simulink model "Dyn_Sim"  (Simulink 9.2)
settings: Solver=VariableStepAuto  StartTime=0.0  StopTime=time  FixedStep=0.1  MaxStep=0.1  RelTol=1e-3  EnableMultiTasking=on
values from neighbouring files (symbols this model uses):
  l10d = -3    [runner_simulation.m]
  l1d = in(15)    [control_law1.m]    (also in runner_simulation.m = 2)
  l2d = 1    [runner_simulation.m]
  l3d = 2    [runner_simulation.m]
  l4d = 1    [runner_simulation.m]
  l5d = 3    [runner_simulation.m]
  l6d = -2    [runner_simulation.m]
  l7d = -2    [runner_simulation.m]
  l8d = 5    [runner_simulation.m]
  l9d = -1    [runner_simulation.m]
  q0 = [10 -18 1*pi/2]'    [runner_simulation.m]
  q0_1 = [22 -18 1*pi/2]'    [runner_simulation.m]
  q0_10 = [14 -18 1*pi/2]'    [runner_simulation.m]
  q0_2 = [18.5 -18 1*pi/2]'    [runner_simulation.m]
  q0_3 = [8 -18 1*pi/2]'    [runner_simulation.m]
  q0_4 = [5 -18 1*pi/2]'    [runner_simulation.m]
  q0_5 = [14 -18 1*pi/2]'    [runner_simulation.m]
  q0_6 = [22 -18 1*pi/2]'    [runner_simulation.m]
  q0_7 = [18.5 -18 1*pi/2]'    [runner_simulation.m]
  q0_8 = [8 -18 1*pi/2]'    [runner_simulation.m]
  q0_9 = [5 -18 1*pi/2]'    [runner_simulation.m]
  sai10_d = 3*pi/6+3*pi/2    (= 6.28318530718)    [runner_simulation.m]
  sai1_d = pi/4    (= 0.785398163397)    [runner_simulation.m]
  sai2_d = 2*pi/4    (= 1.57079632679)    [runner_simulation.m]
  sai3_d = -pi/4    (= -0.785398163397)    [runner_simulation.m]
  sai4_d = -2*pi/4    (= -1.57079632679)    [runner_simulation.m]
  sai5_d = 3*pi/6+3*pi/2    (= 6.28318530718)    [runner_simulation.m]
  sai6_d = pi/4    (= 0.785398163397)    [runner_simulation.m]
  sai7_d = -2*pi/8    (= -0.785398163397)    [runner_simulation.m]
  sai8_d = 3*pi/6+3*pi/2    (= 6.28318530718)    [runner_simulation.m]
  sai9_d = 3*pi/6+3*pi/2    (= 6.28318530718)    [runner_simulation.m]
  u0 = [0.1;0.1;0.1]'    [runner_simulation.m]
  u01 = [0;0;0]'    [runner_simulation.m]
Description:
  | Real-Time Van der Pol Simulation
  | 
  | This demonstration shows a real-time version of the Simulink(R) Van der Pol
  | simulation demo. This model does not need any external signals, so it does
  | not need any data acquisition hardware or driver. This makes the model ideal
  | for first experiments with Real-Time Windows Target(TM), without need to
  | worry about proper I/O hardware configuration.
  | 
  | How to run this demo in Normal Mode:
  | 
  | 1) Double-click the orange button to switch to Normal Mode if needed.
  | 2) Start the real-time execution using Simulation->Start.
  | 3) Observe any missed ticks on the Missed Ticks scope.
  | 
  | How to run this demo in External Mode:
  | 
  | 1) Double-click the orange button to switch to External Mode if needed.
  | 2) Build the model using Tools->Code Generation->Build Model.
  | 3) Connect to the real-time code using Simulation->Connect to target.
  | 4) Start the real-time execution using Simulation->Start real-time code.
  | 5) Missed ticks will be always zero.
settings Model: Creator=The MathWorks Inc.  LastModifiedBy=Rasoul  ExtModeTrigDuration=101
settings DataIOCC: SignalLoggingSaveFormat=Dataset  SignalLoggingName=logsOut
settings OptimizationCC: ExpressionDepthLimit=2147483647  InitFltsAndDblsToZero=on  EfficientMapNaN2IntZero=off
settings DebuggingCC: SignalResolutionControl=TryResolveAllWithWarning  AllowSymbolicDim=off
settings HardwareCC: ProdBitPerPointer=64  ProdBitPerSizeT=64  ProdBitPerPtrDiffT=64  ProdLargestAtomicFloat=Float  ProdIntDivRoundTo=Zero  ProdEndianess=LittleEndian  ProdWordSize=64  ProdHWDeviceType=Intel->x86-64 (Windows64)  TargetBitPerLong=64  TargetBitPerPointer=64  TargetIntDivRoundTo=Zero  TargetEndianess=LittleEndian  TargetWordSize=64  TargetHWDeviceType=Intel->x86-64
settings RTWCC: SystemTargetFile=sldrt.tlc  TemplateMakefile=sldrt.tmf  Description=Simulink Desktop Real-Time  RTWCompilerOptimization=on
settings CodeAppCC: MaxIdLength=95
settings SimulinkDesktopRealTimeCC: TargetPreCompLibLocation=C:\Program Files\MATLAB\R2018b\toolbox\sldrt\lib\win64  TargetLangStandard=C89/C90 (ANSI)  SupportVariableSizeSignals=off  PreserveStateflowLocalDataDimensions=off

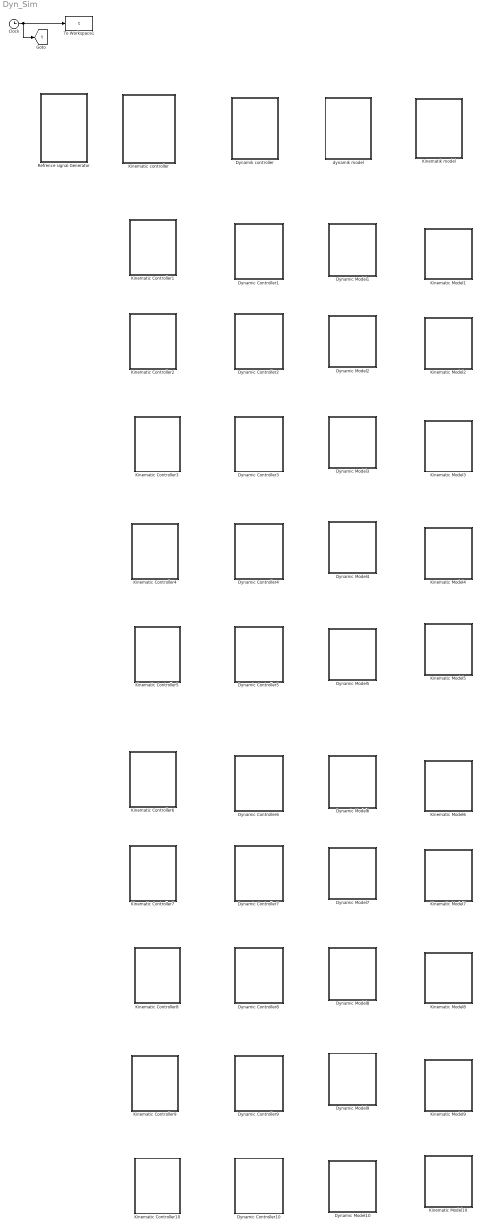
== system Dyn_Sim ==
  Clock : Clock
  Dynamic Controller1 : Subsystem
  Dynamic Controller10 : Subsystem
  Dynamic Controller2 : Subsystem
  Dynamic Controller3 : Subsystem
  Dynamic Controller4 : Subsystem
  Dynamic Controller5 : Subsystem
  Dynamic Controller6 : Subsystem
  Dynamic Controller7 : Subsystem
  Dynamic Controller8 : Subsystem
  Dynamic Controller9 : Subsystem
  Dynamic Model1 : Subsystem
  Dynamic Model10 : Subsystem
  Dynamic Model2 : Subsystem
  Dynamic Model3 : Subsystem
  Dynamic Model4 : Subsystem
  Dynamic Model5 : Subsystem
  Dynamic Model6 : Subsystem
  Dynamic Model7 : Subsystem
  Dynamic Model8 : Subsystem
  Dynamic Model9 : Subsystem
  Dynamik controller : Subsystem
  Kinematic Controller1 : Subsystem
  Kinematic Controller10 : Subsystem
  Kinematic Controller2 : Subsystem
  Kinematic Controller3 : Subsystem
  Kinematic Controller4 : Subsystem
  Kinematic Controller5 : Subsystem
  Kinematic Controller6 : Subsystem
  Kinematic Controller7 : Subsystem
  Kinematic Controller8 : Subsystem
  Kinematic Controller9 : Subsystem
  Kinematic Model1 : Subsystem
  Kinematic Model10 : Subsystem
  Kinematic Model2 : Subsystem
  Kinematic Model3 : Subsystem
  Kinematic Model4 : Subsystem
  Kinematic Model5 : Subsystem
  Kinematic Model6 : Subsystem
  Kinematic Model7 : Subsystem
  Kinematic Model8 : Subsystem
  Kinematic Model9 : Subsystem
  Kinematic controller : Subsystem
  Kinematik model : Subsystem
  "Refrence signal Generator " : Subsystem
  To Workspace1 : ToWorkspace  VariableName=t  SampleTime=-1
  dynamik model : Subsystem
  tag scope: t=global
  wires:
  Clock/1 -> To Workspace1/1, [t]

== system Dyn_Sim/Dynamic Controller1 ==
  Demux1 : Demux  Outputs=2
  Demux2 : Demux  Outputs=3
  Demux4 : Demux  Outputs=3
  Mux4 : Mux  Inputs=3
  Mux7 : Mux
  Mux8 : Mux  Inputs=3
  Scope10 : Scope
  Scope9 : Scope
  To Workspace12 : ToWorkspace  VariableName=tau1  SampleTime=-1
  dynamic_control : MATLABFcn  MATLABFcn=dynamic_control  OutputDimensions=6  OutputSignalType=real
  tag scope: tau1=global
  wires:
  Mux4/1 -> Scope9/1, To Workspace12/1, [tau1]
  Mux7/1 -> dynamic_control/1
  [duc1] -> Mux7/3
  Mux8/1 -> Scope10/1
  Demux4/1 -> Mux4/1
  [t] -> Mux7/4
  [uu1] -> Mux7/1
  [uc1] -> Mux7/2
  dynamic_control/1 -> Demux1/1
  Demux4/2 -> Mux4/2
  Demux1/1 -> Demux4/1
  Demux1/2 -> Demux2/1
  Demux2/1 -> Mux8/1
  Demux2/2 -> Mux8/2
  Demux4/3 -> Mux4/3
  Demux2/3 -> Mux8/3

== system Dyn_Sim/Dynamic Controller10 ==
  Demux1 : Demux  Outputs=2
  Demux2 : Demux  Outputs=3
  Demux4 : Demux  Outputs=3
  Mux4 : Mux  Inputs=3
  Mux7 : Mux
  Mux8 : Mux  Inputs=3
  Scope10 : Scope
  Scope9 : Scope
  To Workspace12 : ToWorkspace  VariableName=tau10  SampleTime=-1
  dynamic_control : MATLABFcn  MATLABFcn=dynamic_control  OutputDimensions=6  OutputSignalType=real
  tag scope: tau10=global
  wires:
  Demux2/3 -> Mux8/3
  Demux4/3 -> Mux4/3
  Demux2/2 -> Mux8/2
  Demux2/1 -> Mux8/1
  Demux1/2 -> Demux2/1
  Demux1/1 -> Demux4/1
  Demux4/2 -> Mux4/2
  dynamic_control/1 -> Demux1/1
  [uc10] -> Mux7/2
  [uu10] -> Mux7/1
  [t] -> Mux7/4
  Demux4/1 -> Mux4/1
  Mux8/1 -> Scope10/1
  [duc10] -> Mux7/3
  Mux7/1 -> dynamic_control/1
  Mux4/1 -> [tau10], To Workspace12/1, Scope9/1

== system Dyn_Sim/Dynamic Controller2 ==
  Demux1 : Demux  Outputs=2
  Demux2 : Demux  Outputs=3
  Demux4 : Demux  Outputs=3
  Mux4 : Mux  Inputs=3
  Mux7 : Mux
  Mux8 : Mux  Inputs=3
  Scope10 : Scope
  Scope9 : Scope
  To Workspace12 : ToWorkspace  VariableName=tau2  SampleTime=-1
  dynamic_control : MATLABFcn  MATLABFcn=dynamic_control  OutputDimensions=6  OutputSignalType=real
  tag scope: tau2=global
  wires:
  Demux2/3 -> Mux8/3
  Demux4/3 -> Mux4/3
  Demux2/1 -> Mux8/1
  Demux4/1 -> Mux4/1
  Mux8/1 -> Scope10/1
  Demux2/2 -> Mux8/2
  [duc2] -> Mux7/3
  dynamic_control/1 -> Demux1/1
  [t] -> Mux7/4
  Demux1/2 -> Demux2/1
  Demux4/2 -> Mux4/2
  [uu2] -> Mux7/1
  Demux1/1 -> Demux4/1
  Mux7/1 -> dynamic_control/1
  [uc2] -> Mux7/2
  Mux4/1 -> [tau2], To Workspace12/1, Scope9/1

== system Dyn_Sim/Dynamic Controller3 ==
  Demux1 : Demux  Outputs=2
  Demux2 : Demux  Outputs=3
  Demux4 : Demux  Outputs=3
  Mux4 : Mux  Inputs=3
  Mux7 : Mux
  Mux8 : Mux  Inputs=3
  Scope10 : Scope
  Scope9 : Scope
  To Workspace12 : ToWorkspace  VariableName=tau3  SampleTime=-1
  dynamic_control : MATLABFcn  MATLABFcn=dynamic_control  OutputDimensions=6  OutputSignalType=real
  tag scope: tau3=global
  wires:
  Mux4/1 -> Scope9/1, To Workspace12/1, [tau3]
  Mux7/1 -> dynamic_control/1
  [duc3] -> Mux7/3
  Mux8/1 -> Scope10/1
  Demux4/1 -> Mux4/1
  [t] -> Mux7/4
  [uu3] -> Mux7/1
  [uc3] -> Mux7/2
  dynamic_control/1 -> Demux1/1
  Demux4/2 -> Mux4/2
  Demux1/1 -> Demux4/1
  Demux1/2 -> Demux2/1
  Demux2/1 -> Mux8/1
  Demux2/2 -> Mux8/2
  Demux4/3 -> Mux4/3
  Demux2/3 -> Mux8/3

== system Dyn_Sim/Dynamic Controller4 ==
  Demux1 : Demux  Outputs=2
  Demux2 : Demux  Outputs=3
  Demux4 : Demux  Outputs=3
  Mux4 : Mux  Inputs=3
  Mux7 : Mux
  Mux8 : Mux  Inputs=3
  Scope10 : Scope
  Scope9 : Scope
  To Workspace12 : ToWorkspace  VariableName=tau4  SampleTime=-1
  dynamic_control : MATLABFcn  MATLABFcn=dynamic_control  OutputDimensions=6  OutputSignalType=real
  tag scope: tau4=global
  wires:
  Mux4/1 -> Scope9/1, To Workspace12/1, [tau4]
  Mux7/1 -> dynamic_control/1
  [duc4] -> Mux7/3
  Mux8/1 -> Scope10/1
  Demux4/1 -> Mux4/1
  [t] -> Mux7/4
  [uu4] -> Mux7/1
  [uc4] -> Mux7/2
  dynamic_control/1 -> Demux1/1
  Demux4/2 -> Mux4/2
  Demux1/1 -> Demux4/1
  Demux1/2 -> Demux2/1
  Demux2/1 -> Mux8/1
  Demux2/2 -> Mux8/2
  Demux4/3 -> Mux4/3
  Demux2/3 -> Mux8/3

== system Dyn_Sim/Dynamic Controller5 ==
  Demux1 : Demux  Outputs=2
  Demux2 : Demux  Outputs=3
  Demux4 : Demux  Outputs=3
  Mux4 : Mux  Inputs=3
  Mux7 : Mux
  Mux8 : Mux  Inputs=3
  Scope10 : Scope
  Scope9 : Scope
  To Workspace12 : ToWorkspace  VariableName=tau5  SampleTime=-1
  dynamic_control : MATLABFcn  MATLABFcn=dynamic_control  OutputDimensions=6  OutputSignalType=real
  tag scope: tau5=global
  wires:
  Mux4/1 -> Scope9/1, To Workspace12/1, [tau5]
  Mux7/1 -> dynamic_control/1
  [duc5] -> Mux7/3
  Mux8/1 -> Scope10/1
  Demux4/1 -> Mux4/1
  [t] -> Mux7/4
  [uu5] -> Mux7/1
  [uc5] -> Mux7/2
  dynamic_control/1 -> Demux1/1
  Demux4/2 -> Mux4/2
  Demux1/1 -> Demux4/1
  Demux1/2 -> Demux2/1
  Demux2/1 -> Mux8/1
  Demux2/2 -> Mux8/2
  Demux4/3 -> Mux4/3
  Demux2/3 -> Mux8/3

== system Dyn_Sim/Dynamic Controller6 ==
  Demux1 : Demux  Outputs=2
  Demux2 : Demux  Outputs=3
  Demux4 : Demux  Outputs=3
  Mux4 : Mux  Inputs=3
  Mux7 : Mux
  Mux8 : Mux  Inputs=3
  Scope10 : Scope
  Scope9 : Scope
  To Workspace12 : ToWorkspace  VariableName=tau6  SampleTime=-1
  dynamic_control : MATLABFcn  MATLABFcn=dynamic_control  OutputDimensions=6  OutputSignalType=real
  tag scope: tau6=global
  wires:
  Demux2/3 -> Mux8/3
  Demux4/3 -> Mux4/3
  Demux2/2 -> Mux8/2
  Demux2/1 -> Mux8/1
  Demux1/2 -> Demux2/1
  Demux1/1 -> Demux4/1
  Demux4/2 -> Mux4/2
  dynamic_control/1 -> Demux1/1
  [uc6] -> Mux7/2
  [uu6] -> Mux7/1
  [t] -> Mux7/4
  Demux4/1 -> Mux4/1
  Mux8/1 -> Scope10/1
  [duc6] -> Mux7/3
  Mux7/1 -> dynamic_control/1
  Mux4/1 -> [tau6], To Workspace12/1, Scope9/1

== system Dyn_Sim/Dynamic Controller7 ==
  Demux1 : Demux  Outputs=2
  Demux2 : Demux  Outputs=3
  Demux4 : Demux  Outputs=3
  Mux4 : Mux  Inputs=3
  Mux7 : Mux
  Mux8 : Mux  Inputs=3
  Scope10 : Scope
  Scope9 : Scope
  To Workspace12 : ToWorkspace  VariableName=tau7  SampleTime=-1
  dynamic_control : MATLABFcn  MATLABFcn=dynamic_control  OutputDimensions=6  OutputSignalType=real
  tag scope: tau7=global
  wires:
  Mux4/1 -> Scope9/1, To Workspace12/1, [tau7]
  [uc7] -> Mux7/2
  Mux7/1 -> dynamic_control/1
  Demux1/1 -> Demux4/1
  [uu7] -> Mux7/1
  Demux4/2 -> Mux4/2
  Demux1/2 -> Demux2/1
  [t] -> Mux7/4
  dynamic_control/1 -> Demux1/1
  [duc7] -> Mux7/3
  Demux2/2 -> Mux8/2
  Mux8/1 -> Scope10/1
  Demux4/1 -> Mux4/1
  Demux2/1 -> Mux8/1
  Demux4/3 -> Mux4/3
  Demux2/3 -> Mux8/3

== system Dyn_Sim/Dynamic Controller8 ==
  Demux1 : Demux  Outputs=2
  Demux2 : Demux  Outputs=3
  Demux4 : Demux  Outputs=3
  Mux4 : Mux  Inputs=3
  Mux7 : Mux
  Mux8 : Mux  Inputs=3
  Scope10 : Scope
  Scope9 : Scope
  To Workspace12 : ToWorkspace  VariableName=tau8  SampleTime=-1
  dynamic_control : MATLABFcn  MATLABFcn=dynamic_control  OutputDimensions=6  OutputSignalType=real
  tag scope: tau8=global
  wires:
  Demux2/3 -> Mux8/3
  Demux4/3 -> Mux4/3
  Demux2/2 -> Mux8/2
  Demux2/1 -> Mux8/1
  Demux1/2 -> Demux2/1
  Demux1/1 -> Demux4/1
  Demux4/2 -> Mux4/2
  dynamic_control/1 -> Demux1/1
  [uc8] -> Mux7/2
  [uu8] -> Mux7/1
  [t] -> Mux7/4
  Demux4/1 -> Mux4/1
  Mux8/1 -> Scope10/1
  [duc8] -> Mux7/3
  Mux7/1 -> dynamic_control/1
  Mux4/1 -> [tau8], To Workspace12/1, Scope9/1

== system Dyn_Sim/Dynamic Controller9 ==
  Demux1 : Demux  Outputs=2
  Demux2 : Demux  Outputs=3
  Demux4 : Demux  Outputs=3
  Mux4 : Mux  Inputs=3
  Mux7 : Mux
  Mux8 : Mux  Inputs=3
  Scope10 : Scope
  Scope9 : Scope
  To Workspace12 : ToWorkspace  VariableName=tau9  SampleTime=-1
  dynamic_control : MATLABFcn  MATLABFcn=dynamic_control  OutputDimensions=6  OutputSignalType=real
  tag scope: tau9=global
  wires:
  Demux2/3 -> Mux8/3
  Demux4/3 -> Mux4/3
  Demux2/2 -> Mux8/2
  Demux2/1 -> Mux8/1
  Demux1/2 -> Demux2/1
  Demux1/1 -> Demux4/1
  Demux4/2 -> Mux4/2
  dynamic_control/1 -> Demux1/1
  [uc9] -> Mux7/2
  [uu9] -> Mux7/1
  [t] -> Mux7/4
  Demux4/1 -> Mux4/1
  Mux8/1 -> Scope10/1
  [duc9] -> Mux7/3
  Mux7/1 -> dynamic_control/1
  Mux4/1 -> [tau9], To Workspace12/1, Scope9/1

== system Dyn_Sim/Dynamic Model1 ==
  Integrator2 : Integrator  InitialCondition=u01
  Mux9 : Mux  Inputs=3
  To Workspace11 : ToWorkspace  VariableName=uu1  SampleTime=-1
  dynamic_model : MATLABFcn  MATLABFcn=dynamic_model  OutputDimensions=3  OutputSignalType=real
  tag scope: uu1=global
  wires:
  [tau1] -> Mux9/2
  [uu1] -> Mux9/1
  dynamic_model/1 -> Integrator2/1
  Mux9/1 -> dynamic_model/1
  [t] -> Mux9/3
  Integrator2/1 -> [uu1], To Workspace11/1

== system Dyn_Sim/Dynamic Model10 ==
  Integrator2 : Integrator  InitialCondition=u01
  Mux9 : Mux  Inputs=3
  To Workspace11 : ToWorkspace  VariableName=uu10  SampleTime=-1
  dynamic_model : MATLABFcn  MATLABFcn=dynamic_model  OutputDimensions=3  OutputSignalType=real
  tag scope: uu10=global
  wires:
  Integrator2/1 -> To Workspace11/1, [uu10]
  [t] -> Mux9/3
  Mux9/1 -> dynamic_model/1
  dynamic_model/1 -> Integrator2/1
  [uu10] -> Mux9/1
  [tau10] -> Mux9/2

== system Dyn_Sim/Dynamic Model2 ==
  Integrator2 : Integrator  InitialCondition=u01
  Mux9 : Mux  Inputs=3
  To Workspace11 : ToWorkspace  VariableName=uu2  SampleTime=-1
  dynamic_model : MATLABFcn  MATLABFcn=dynamic_model  OutputDimensions=3  OutputSignalType=real
  tag scope: uu2=global
  wires:
  Mux9/1 -> dynamic_model/1
  [tau2] -> Mux9/2
  dynamic_model/1 -> Integrator2/1
  Integrator2/1 -> To Workspace11/1, [uu2]
  [t] -> Mux9/3
  [uu2] -> Mux9/1

== system Dyn_Sim/Dynamic Model3 ==
  Integrator2 : Integrator  InitialCondition=u01
  Mux9 : Mux  Inputs=3
  To Workspace11 : ToWorkspace  VariableName=uu3  SampleTime=-1
  dynamic_model : MATLABFcn  MATLABFcn=dynamic_model  OutputDimensions=3  OutputSignalType=real
  tag scope: uu3=global
  wires:
  [tau3] -> Mux9/2
  [uu3] -> Mux9/1
  dynamic_model/1 -> Integrator2/1
  Mux9/1 -> dynamic_model/1
  [t] -> Mux9/3
  Integrator2/1 -> [uu3], To Workspace11/1

== system Dyn_Sim/Dynamic Model4 ==
  Integrator2 : Integrator  InitialCondition=u01
  Mux9 : Mux  Inputs=3
  To Workspace11 : ToWorkspace  VariableName=uu4  SampleTime=-1
  dynamic_model : MATLABFcn  MATLABFcn=dynamic_model  OutputDimensions=3  OutputSignalType=real
  tag scope: uu4=global
  wires:
  [tau4] -> Mux9/2
  [uu4] -> Mux9/1
  dynamic_model/1 -> Integrator2/1
  Mux9/1 -> dynamic_model/1
  [t] -> Mux9/3
  Integrator2/1 -> [uu4], To Workspace11/1

== system Dyn_Sim/Dynamic Model5 ==
  Integrator2 : Integrator  InitialCondition=u01
  Mux9 : Mux  Inputs=3
  To Workspace11 : ToWorkspace  VariableName=uu5  SampleTime=-1
  dynamic_model : MATLABFcn  MATLABFcn=dynamic_model  OutputDimensions=3  OutputSignalType=real
  tag scope: uu5=global
  wires:
  [tau5] -> Mux9/2
  [uu5] -> Mux9/1
  dynamic_model/1 -> Integrator2/1
  Mux9/1 -> dynamic_model/1
  [t] -> Mux9/3
  Integrator2/1 -> [uu5], To Workspace11/1

== system Dyn_Sim/Dynamic Model6 ==
  Integrator2 : Integrator  InitialCondition=u01
  Mux9 : Mux  Inputs=3
  To Workspace11 : ToWorkspace  VariableName=uu6  SampleTime=-1
  dynamic_model : MATLABFcn  MATLABFcn=dynamic_model  OutputDimensions=3  OutputSignalType=real
  tag scope: uu6=global
  wires:
  Integrator2/1 -> To Workspace11/1, [uu6]
  [t] -> Mux9/3
  Mux9/1 -> dynamic_model/1
  dynamic_model/1 -> Integrator2/1
  [uu6] -> Mux9/1
  [tau6] -> Mux9/2

== system Dyn_Sim/Dynamic Model7 ==
  Integrator2 : Integrator  InitialCondition=u01
  Mux9 : Mux  Inputs=3
  To Workspace11 : ToWorkspace  VariableName=uu7  SampleTime=-1
  dynamic_model : MATLABFcn  MATLABFcn=dynamic_model  OutputDimensions=3  OutputSignalType=real
  tag scope: uu7=global
  wires:
  [uu7] -> Mux9/1
  [t] -> Mux9/3
  Integrator2/1 -> [uu7], To Workspace11/1
  dynamic_model/1 -> Integrator2/1
  [tau7] -> Mux9/2
  Mux9/1 -> dynamic_model/1

== system Dyn_Sim/Dynamic Model8 ==
  Integrator2 : Integrator  InitialCondition=u01
  Mux9 : Mux  Inputs=3
  To Workspace11 : ToWorkspace  VariableName=uu8  SampleTime=-1
  dynamic_model : MATLABFcn  MATLABFcn=dynamic_model  OutputDimensions=3  OutputSignalType=real
  tag scope: uu8=global
  wires:
  Integrator2/1 -> To Workspace11/1, [uu8]
  [t] -> Mux9/3
  Mux9/1 -> dynamic_model/1
  dynamic_model/1 -> Integrator2/1
  [uu8] -> Mux9/1
  [tau8] -> Mux9/2

== system Dyn_Sim/Dynamic Model9 ==
  Integrator2 : Integrator  InitialCondition=u01
  Mux9 : Mux  Inputs=3
  To Workspace11 : ToWorkspace  VariableName=uu9  SampleTime=-1
  dynamic_model : MATLABFcn  MATLABFcn=dynamic_model  OutputDimensions=3  OutputSignalType=real
  tag scope: uu9=global
  wires:
  Integrator2/1 -> To Workspace11/1, [uu9]
  [t] -> Mux9/3
  Mux9/1 -> dynamic_model/1
  dynamic_model/1 -> Integrator2/1
  [uu9] -> Mux9/1
  [tau9] -> Mux9/2

== system Dyn_Sim/Dynamik controller ==
  Demux4 : Demux  Outputs=6
  Mux4 : Mux  Inputs=3
  Mux7 : Mux
  Mux8 : Mux  Inputs=3
  Scope10 : Scope
  Scope9 : Scope
  To Workspace12 : ToWorkspace  VariableName=tau  SampleTime=-1
  dynamic_control : MATLABFcn  MATLABFcn=dynamic_control  OutputDimensions=6  OutputSignalType=real
  tag scope: tau=global
  wires:
  Demux4/6 -> Mux8/3
  Demux4/5 -> Mux8/2
  Demux4/3 -> Mux4/3
  Mux4/1 -> To Workspace12/1, Scope9/1, [tau]
  dynamic_control/1 -> Demux4/1
  [uu] -> Mux7/1
  Mux8/1 -> Scope10/1
  Demux4/4 -> Mux8/1
  [duc] -> Mux7/3
  [uc] -> Mux7/2
  Demux4/1 -> Mux4/1
  Demux4/2 -> Mux4/2
  Mux7/1 -> dynamic_control/1
  [t] -> Mux7/4

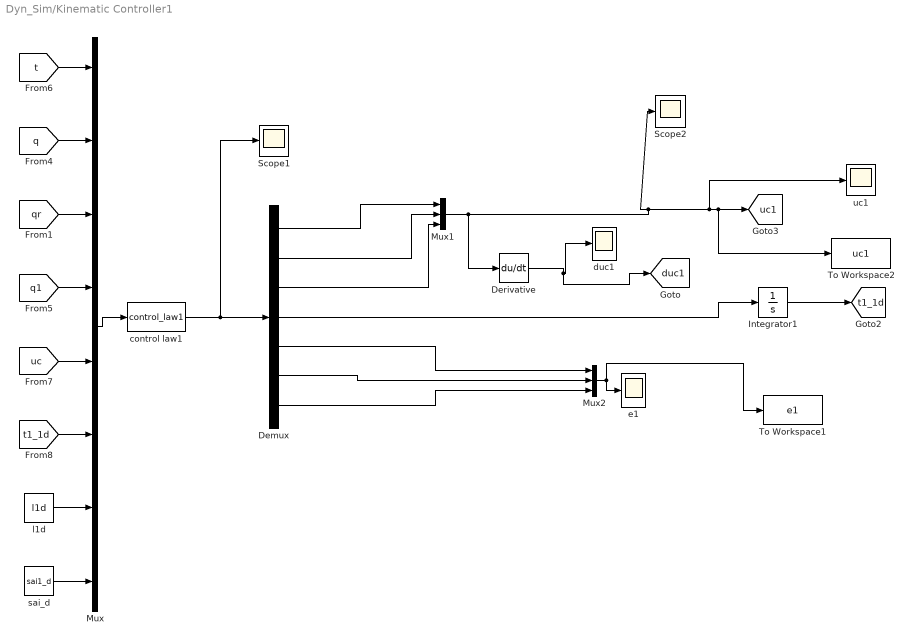
== system Dyn_Sim/Kinematic Controller1 ==
  Demux : Demux  Outputs=7
  Derivative : Derivative
  Integrator1 : Integrator  InitialCondition=pi/2
  Mux : Mux  Inputs=8
  Mux1 : Mux  Inputs=3
  Mux2 : Mux  Inputs=3
  Scope1 : Scope
  Scope2 : Scope
  To Workspace1 : ToWorkspace  VariableName=e1  SampleTime=-1
  To Workspace2 : ToWorkspace  VariableName=uc1  SampleTime=-1
  control law1 : MATLABFcn  MATLABFcn=control_law1  OutputDimensions=7  OutputSignalType=real
  duc1 : Scope
  e1 : Scope
  l1d : Constant  Value=l1d
  sai_d : Constant  Value=sai1_d
  uc1 : Scope
  tag scope: duc1=global, t1_1d=global, uc1=global
  wires:
  control law1/1 -> Scope1/1, Demux/1
  Mux/1 -> control law1/1
  Integrator1/1 -> [t1_1d]
  Mux1/1 -> Derivative/1, uc1/1, To Workspace2/1, [uc1], Scope2/1
  Demux/1 -> Mux1/1
  Demux/2 -> Mux1/2
  Mux2/1 -> e1/1, To Workspace1/1
  Derivative/1 -> [duc1], duc1/1
  [uc] -> Mux/5
  [q1] -> Mux/4
  [qr] -> Mux/3
  [q] -> Mux/2
  [t] -> Mux/1
  [t1_1d] -> Mux/6
  l1d/1 -> Mux/7
  sai_d/1 -> Mux/8
  Demux/3 -> Mux1/3
  Demux/4 -> Integrator1/1
  Demux/5 -> Mux2/1
  Demux/6 -> Mux2/2
  Demux/7 -> Mux2/3

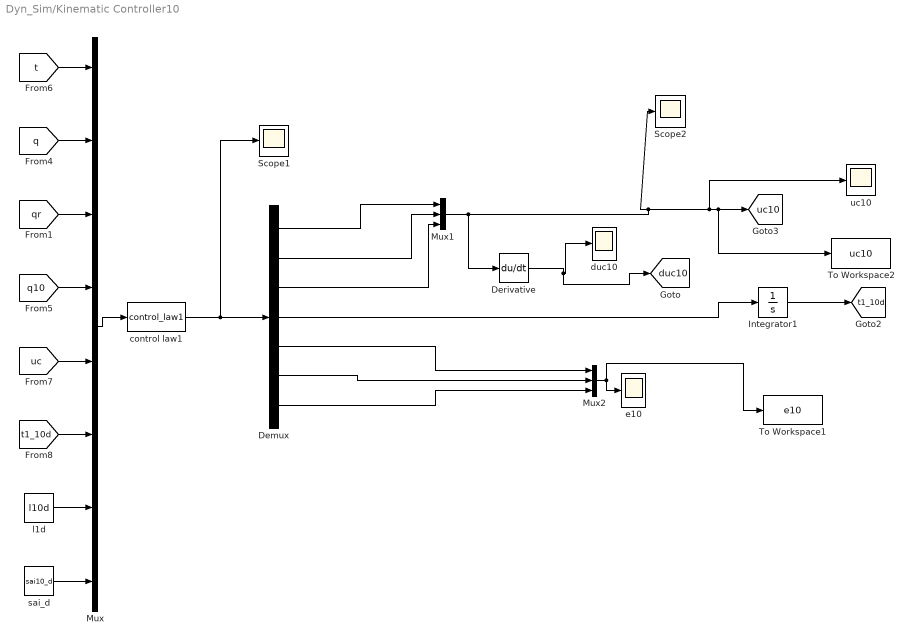
== system Dyn_Sim/Kinematic Controller10 ==
  Demux : Demux  Outputs=7
  Derivative : Derivative
  Integrator1 : Integrator  InitialCondition=pi/2
  Mux : Mux  Inputs=8
  Mux1 : Mux  Inputs=3
  Mux2 : Mux  Inputs=3
  Scope1 : Scope
  Scope2 : Scope
  To Workspace1 : ToWorkspace  VariableName=e10  SampleTime=-1
  To Workspace2 : ToWorkspace  VariableName=uc10  SampleTime=-1
  control law1 : MATLABFcn  MATLABFcn=control_law1  OutputDimensions=7  OutputSignalType=real
  duc10 : Scope
  "e10 " : Scope
  l1d : Constant  Value=l10d
  sai_d : Constant  Value=sai10_d
  uc10 : Scope
  tag scope: duc10=global, t1_10d=global, uc10=global
  wires:
  Demux/7 -> Mux2/3
  Demux/6 -> Mux2/2
  Demux/5 -> Mux2/1
  Demux/4 -> Integrator1/1
  Demux/3 -> Mux1/3
  sai_d/1 -> Mux/8
  l1d/1 -> Mux/7
  [t1_10d] -> Mux/6
  [t] -> Mux/1
  [q] -> Mux/2
  [qr] -> Mux/3
  [q10] -> Mux/4
  [uc] -> Mux/5
  Derivative/1 -> duc10/1, [duc10]
  Mux2/1 -> To Workspace1/1, "e10 "/1
  Demux/2 -> Mux1/2
  Demux/1 -> Mux1/1
  Mux1/1 -> Scope2/1, [uc10], To Workspace2/1, uc10/1, Derivative/1
  Integrator1/1 -> [t1_10d]
  Mux/1 -> control law1/1
  control law1/1 -> Demux/1, Scope1/1

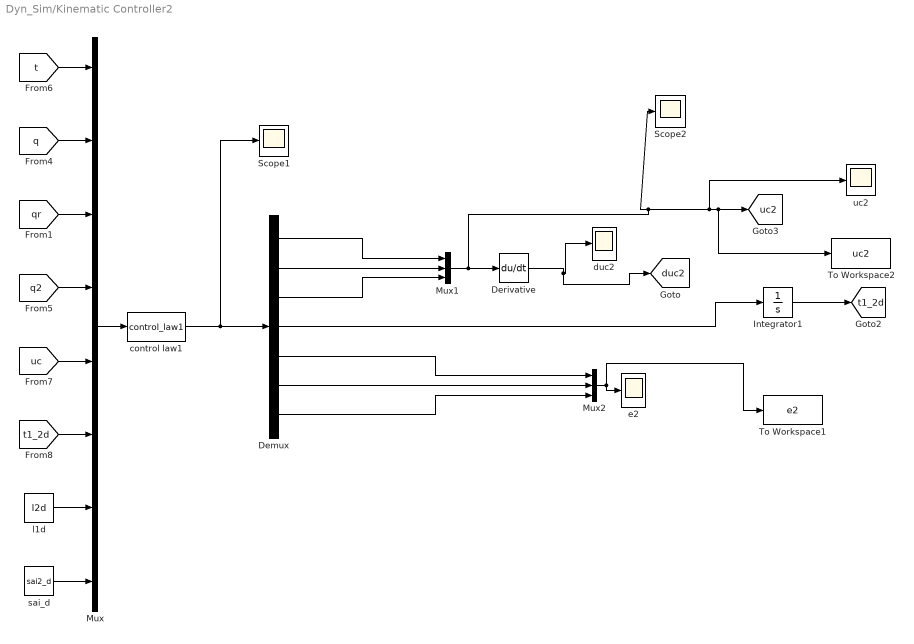
== system Dyn_Sim/Kinematic Controller2 ==
  Demux : Demux  Outputs=7
  Derivative : Derivative
  Integrator1 : Integrator  InitialCondition=pi/2
  Mux : Mux  Inputs=8
  Mux1 : Mux  Inputs=3
  Mux2 : Mux  Inputs=3
  Scope1 : Scope
  Scope2 : Scope
  To Workspace1 : ToWorkspace  VariableName=e2  SampleTime=-1
  To Workspace2 : ToWorkspace  VariableName=uc2  SampleTime=-1
  control law1 : MATLABFcn  MATLABFcn=control_law1  OutputDimensions=7  OutputSignalType=real
  duc2 : Scope
  e2 : Scope
  l1d : Constant  Value=l2d
  sai_d : Constant  Value=sai2_d
  uc2 : Scope
  tag scope: duc2=global, t1_2d=global, uc2=global
  wires:
  Mux/1 -> control law1/1
  control law1/1 -> Demux/1, Scope1/1
  Mux1/1 -> Scope2/1, [uc2], To Workspace2/1, uc2/1, Derivative/1
  Integrator1/1 -> [t1_2d]
  Demux/1 -> Mux1/1
  [q2] -> Mux/4
  Demux/2 -> Mux1/2
  Derivative/1 -> duc2/1, [duc2]
  [t] -> Mux/1
  [uc] -> Mux/5
  [qr] -> Mux/3
  [q] -> Mux/2
  Mux2/1 -> To Workspace1/1, e2/1
  [t1_2d] -> Mux/6
  l1d/1 -> Mux/7
  sai_d/1 -> Mux/8
  Demux/3 -> Mux1/3
  Demux/4 -> Integrator1/1
  Demux/5 -> Mux2/1
  Demux/6 -> Mux2/2
  Demux/7 -> Mux2/3

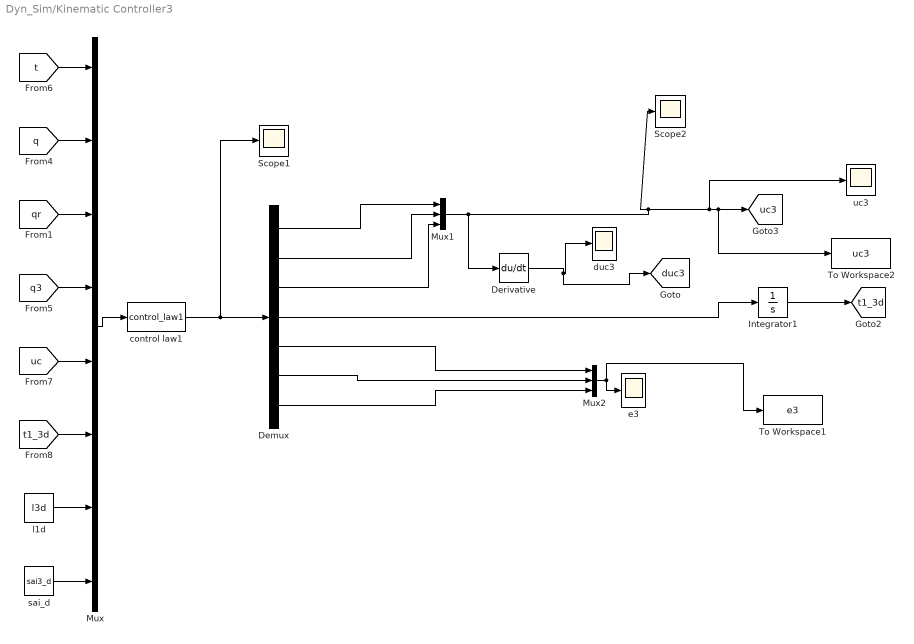
== system Dyn_Sim/Kinematic Controller3 ==
  Demux : Demux  Outputs=7
  Derivative : Derivative
  Integrator1 : Integrator  InitialCondition=pi/2
  Mux : Mux  Inputs=8
  Mux1 : Mux  Inputs=3
  Mux2 : Mux  Inputs=3
  Scope1 : Scope
  Scope2 : Scope
  To Workspace1 : ToWorkspace  VariableName=e3  SampleTime=-1
  To Workspace2 : ToWorkspace  VariableName=uc3  SampleTime=-1
  control law1 : MATLABFcn  MATLABFcn=control_law1  OutputDimensions=7  OutputSignalType=real
  duc3 : Scope
  e3 : Scope
  l1d : Constant  Value=l3d
  sai_d : Constant  Value=sai3_d
  uc3 : Scope
  tag scope: duc3=global, t1_3d=global, uc3=global
  wires:
  control law1/1 -> Scope1/1, Demux/1
  Mux/1 -> control law1/1
  Integrator1/1 -> [t1_3d]
  Mux1/1 -> Derivative/1, uc3/1, To Workspace2/1, [uc3], Scope2/1
  Demux/1 -> Mux1/1
  Demux/2 -> Mux1/2
  Mux2/1 -> e3/1, To Workspace1/1
  Derivative/1 -> [duc3], duc3/1
  [uc] -> Mux/5
  [q3] -> Mux/4
  [qr] -> Mux/3
  [q] -> Mux/2
  [t] -> Mux/1
  [t1_3d] -> Mux/6
  l1d/1 -> Mux/7
  sai_d/1 -> Mux/8
  Demux/3 -> Mux1/3
  Demux/4 -> Integrator1/1
  Demux/5 -> Mux2/1
  Demux/6 -> Mux2/2
  Demux/7 -> Mux2/3

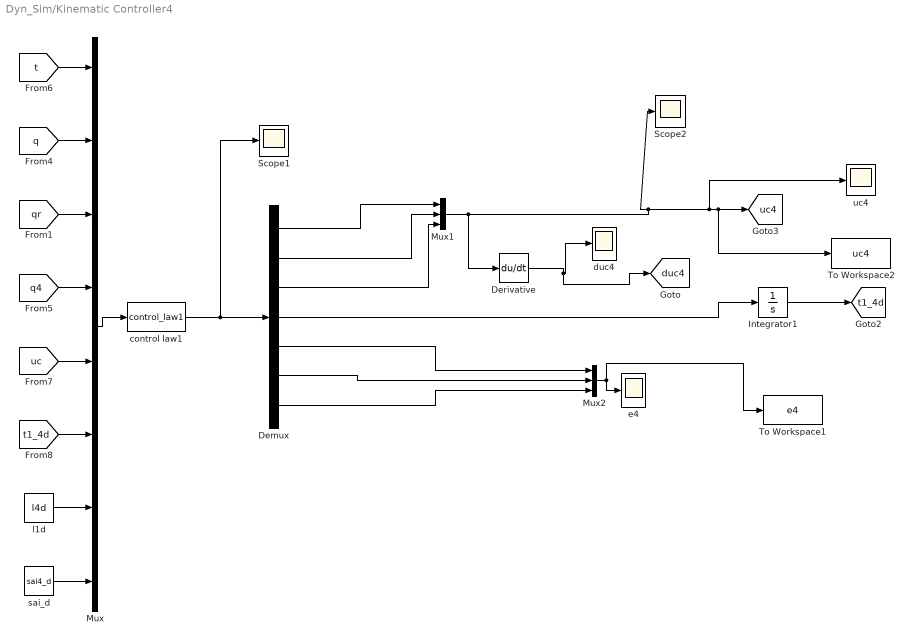
== system Dyn_Sim/Kinematic Controller4 ==
  Demux : Demux  Outputs=7
  Derivative : Derivative
  Integrator1 : Integrator  InitialCondition=pi/2
  Mux : Mux  Inputs=8
  Mux1 : Mux  Inputs=3
  Mux2 : Mux  Inputs=3
  Scope1 : Scope
  Scope2 : Scope
  To Workspace1 : ToWorkspace  VariableName=e4  SampleTime=-1
  To Workspace2 : ToWorkspace  VariableName=uc4  SampleTime=-1
  control law1 : MATLABFcn  MATLABFcn=control_law1  OutputDimensions=7  OutputSignalType=real
  duc4 : Scope
  e4 : Scope
  l1d : Constant  Value=l4d
  sai_d : Constant  Value=sai4_d
  uc4 : Scope
  tag scope: duc4=global, t1_4d=global, uc4=global
  wires:
  control law1/1 -> Scope1/1, Demux/1
  Mux/1 -> control law1/1
  Integrator1/1 -> [t1_4d]
  Mux1/1 -> Derivative/1, uc4/1, To Workspace2/1, [uc4], Scope2/1
  Demux/1 -> Mux1/1
  Demux/2 -> Mux1/2
  Mux2/1 -> e4/1, To Workspace1/1
  Derivative/1 -> [duc4], duc4/1
  [uc] -> Mux/5
  [q4] -> Mux/4
  [qr] -> Mux/3
  [q] -> Mux/2
  [t] -> Mux/1
  [t1_4d] -> Mux/6
  l1d/1 -> Mux/7
  sai_d/1 -> Mux/8
  Demux/3 -> Mux1/3
  Demux/4 -> Integrator1/1
  Demux/5 -> Mux2/1
  Demux/6 -> Mux2/2
  Demux/7 -> Mux2/3

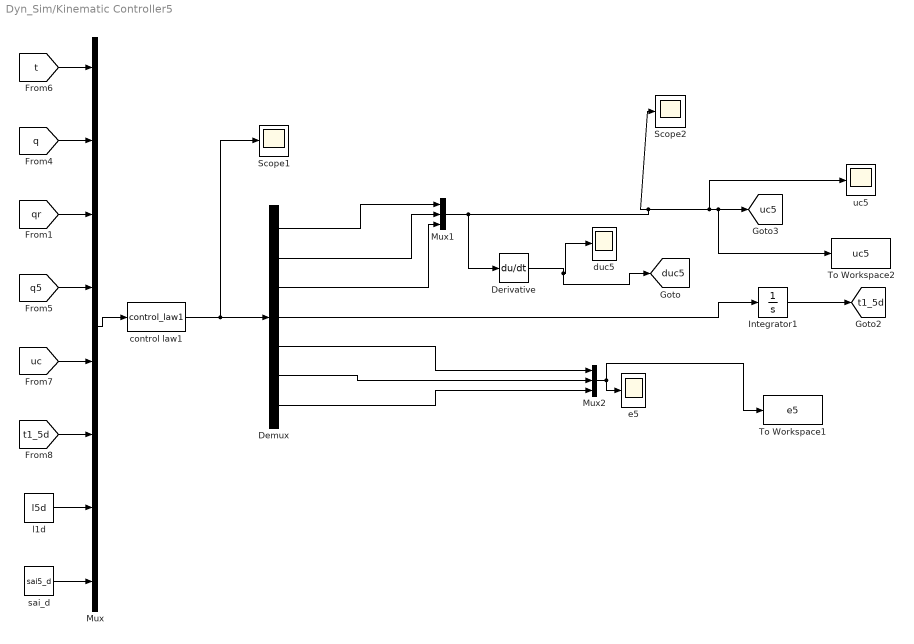
== system Dyn_Sim/Kinematic Controller5 ==
  Demux : Demux  Outputs=7
  Derivative : Derivative
  Integrator1 : Integrator  InitialCondition=pi/2
  Mux : Mux  Inputs=8
  Mux1 : Mux  Inputs=3
  Mux2 : Mux  Inputs=3
  Scope1 : Scope
  Scope2 : Scope
  To Workspace1 : ToWorkspace  VariableName=e5  SampleTime=-1
  To Workspace2 : ToWorkspace  VariableName=uc5  SampleTime=-1
  control law1 : MATLABFcn  MATLABFcn=control_law1  OutputDimensions=7  OutputSignalType=real
  duc5 : Scope
  "e5 " : Scope
  l1d : Constant  Value=l5d
  sai_d : Constant  Value=sai5_d
  uc5 : Scope
  tag scope: duc5=global, t1_5d=global, uc5=global
  wires:
  control law1/1 -> Scope1/1, Demux/1
  Mux/1 -> control law1/1
  Integrator1/1 -> [t1_5d]
  Mux1/1 -> Derivative/1, uc5/1, To Workspace2/1, [uc5], Scope2/1
  Demux/1 -> Mux1/1
  Demux/2 -> Mux1/2
  Mux2/1 -> "e5 "/1, To Workspace1/1
  Derivative/1 -> [duc5], duc5/1
  [uc] -> Mux/5
  [q5] -> Mux/4
  [qr] -> Mux/3
  [q] -> Mux/2
  [t] -> Mux/1
  [t1_5d] -> Mux/6
  l1d/1 -> Mux/7
  sai_d/1 -> Mux/8
  Demux/3 -> Mux1/3
  Demux/4 -> Integrator1/1
  Demux/5 -> Mux2/1
  Demux/6 -> Mux2/2
  Demux/7 -> Mux2/3

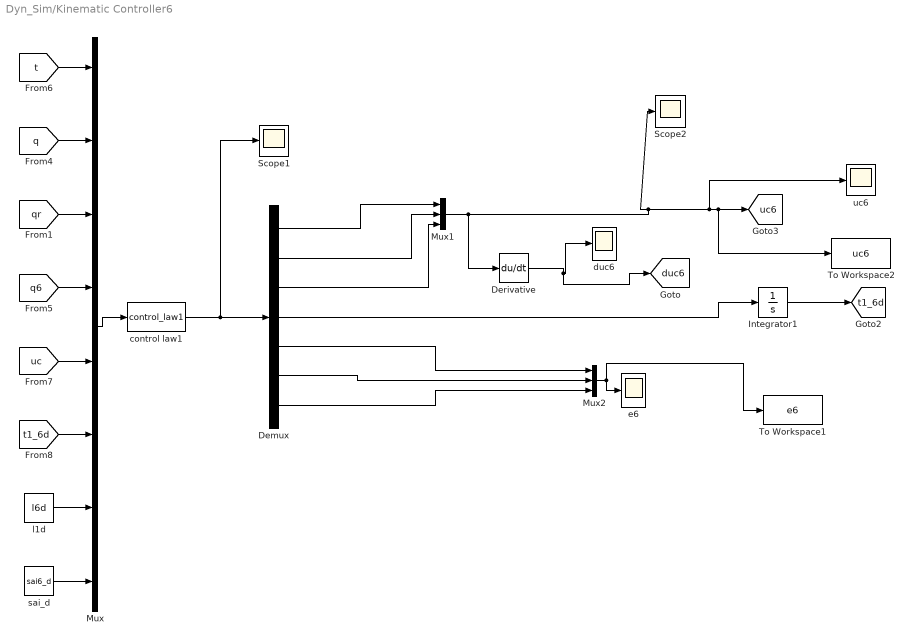
== system Dyn_Sim/Kinematic Controller6 ==
  Demux : Demux  Outputs=7
  Derivative : Derivative
  Integrator1 : Integrator  InitialCondition=pi/2
  Mux : Mux  Inputs=8
  Mux1 : Mux  Inputs=3
  Mux2 : Mux  Inputs=3
  Scope1 : Scope
  Scope2 : Scope
  To Workspace1 : ToWorkspace  VariableName=e6  SampleTime=-1
  To Workspace2 : ToWorkspace  VariableName=uc6  SampleTime=-1
  control law1 : MATLABFcn  MATLABFcn=control_law1  OutputDimensions=7  OutputSignalType=real
  duc6 : Scope
  e6 : Scope
  l1d : Constant  Value=l6d
  sai_d : Constant  Value=sai6_d
  uc6 : Scope
  tag scope: duc6=global, t1_6d=global, uc6=global
  wires:
  Demux/7 -> Mux2/3
  Demux/6 -> Mux2/2
  Demux/5 -> Mux2/1
  Demux/4 -> Integrator1/1
  Demux/3 -> Mux1/3
  sai_d/1 -> Mux/8
  l1d/1 -> Mux/7
  [t1_6d] -> Mux/6
  [t] -> Mux/1
  [q] -> Mux/2
  [qr] -> Mux/3
  [q6] -> Mux/4
  [uc] -> Mux/5
  Derivative/1 -> duc6/1, [duc6]
  Mux2/1 -> To Workspace1/1, e6/1
  Demux/2 -> Mux1/2
  Demux/1 -> Mux1/1
  Mux1/1 -> Scope2/1, [uc6], To Workspace2/1, uc6/1, Derivative/1
  Integrator1/1 -> [t1_6d]
  Mux/1 -> control law1/1
  control law1/1 -> Demux/1, Scope1/1

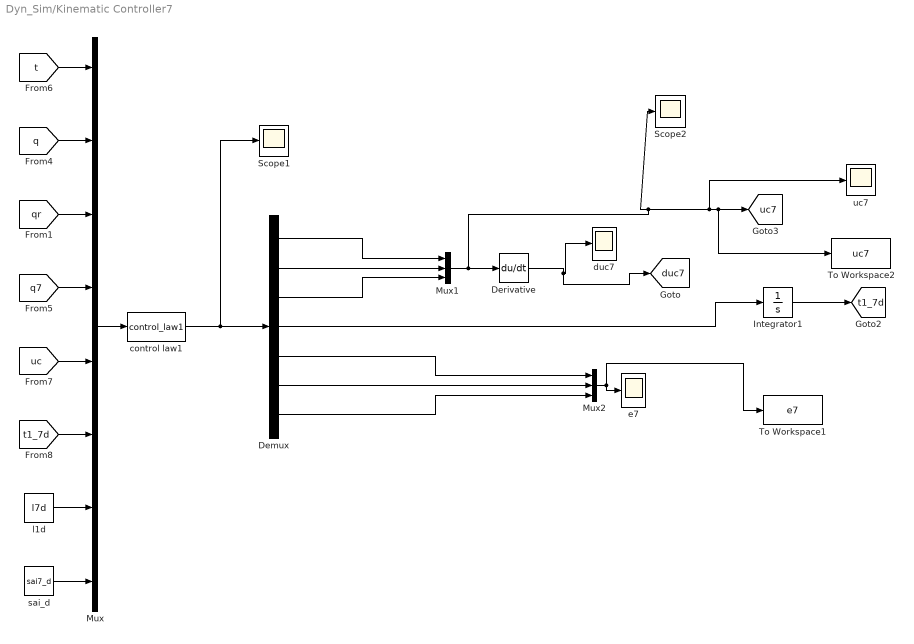
== system Dyn_Sim/Kinematic Controller7 ==
  Demux : Demux  Outputs=7
  Derivative : Derivative
  Integrator1 : Integrator  InitialCondition=pi/2
  Mux : Mux  Inputs=8
  Mux1 : Mux  Inputs=3
  Mux2 : Mux  Inputs=3
  Scope1 : Scope
  Scope2 : Scope
  To Workspace1 : ToWorkspace  VariableName=e7  SampleTime=-1
  To Workspace2 : ToWorkspace  VariableName=uc7  SampleTime=-1
  control law1 : MATLABFcn  MATLABFcn=control_law1  OutputDimensions=7  OutputSignalType=real
  duc7 : Scope
  e7 : Scope
  l1d : Constant  Value=l7d
  sai_d : Constant  Value=sai7_d
  uc7 : Scope
  tag scope: duc7=global, t1_7d=global, uc7=global
  wires:
  Demux/7 -> Mux2/3
  Demux/6 -> Mux2/2
  Demux/5 -> Mux2/1
  Demux/4 -> Integrator1/1
  Demux/3 -> Mux1/3
  sai_d/1 -> Mux/8
  l1d/1 -> Mux/7
  [t1_7d] -> Mux/6
  Mux2/1 -> e7/1, To Workspace1/1
  [q] -> Mux/2
  [qr] -> Mux/3
  [uc] -> Mux/5
  [t] -> Mux/1
  Derivative/1 -> [duc7], duc7/1
  Demux/2 -> Mux1/2
  [q7] -> Mux/4
  Demux/1 -> Mux1/1
  Integrator1/1 -> [t1_7d]
  Mux1/1 -> Derivative/1, uc7/1, To Workspace2/1, [uc7], Scope2/1
  control law1/1 -> Scope1/1, Demux/1
  Mux/1 -> control law1/1

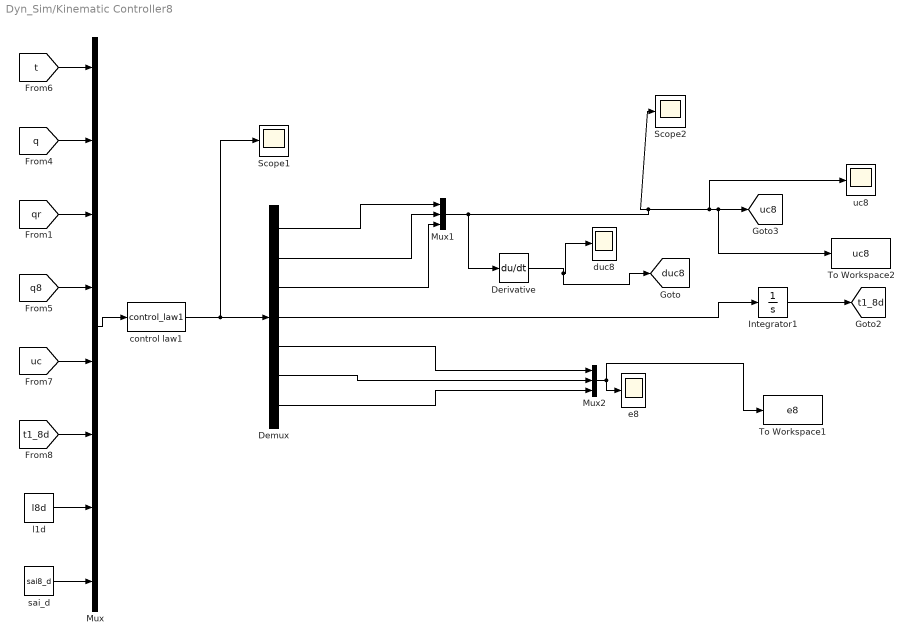
== system Dyn_Sim/Kinematic Controller8 ==
  Demux : Demux  Outputs=7
  Derivative : Derivative
  Integrator1 : Integrator  InitialCondition=pi/2
  Mux : Mux  Inputs=8
  Mux1 : Mux  Inputs=3
  Mux2 : Mux  Inputs=3
  Scope1 : Scope
  Scope2 : Scope
  To Workspace1 : ToWorkspace  VariableName=e8  SampleTime=-1
  To Workspace2 : ToWorkspace  VariableName=uc8  SampleTime=-1
  control law1 : MATLABFcn  MATLABFcn=control_law1  OutputDimensions=7  OutputSignalType=real
  duc8 : Scope
  e8 : Scope
  l1d : Constant  Value=l8d
  sai_d : Constant  Value=sai8_d
  uc8 : Scope
  tag scope: duc8=global, t1_8d=global, uc8=global
  wires:
  Demux/7 -> Mux2/3
  Demux/6 -> Mux2/2
  Demux/5 -> Mux2/1
  Demux/4 -> Integrator1/1
  Demux/3 -> Mux1/3
  sai_d/1 -> Mux/8
  l1d/1 -> Mux/7
  [t1_8d] -> Mux/6
  [t] -> Mux/1
  [q] -> Mux/2
  [qr] -> Mux/3
  [q8] -> Mux/4
  [uc] -> Mux/5
  Derivative/1 -> duc8/1, [duc8]
  Mux2/1 -> To Workspace1/1, e8/1
  Demux/2 -> Mux1/2
  Demux/1 -> Mux1/1
  Mux1/1 -> Scope2/1, [uc8], To Workspace2/1, uc8/1, Derivative/1
  Integrator1/1 -> [t1_8d]
  Mux/1 -> control law1/1
  control law1/1 -> Demux/1, Scope1/1

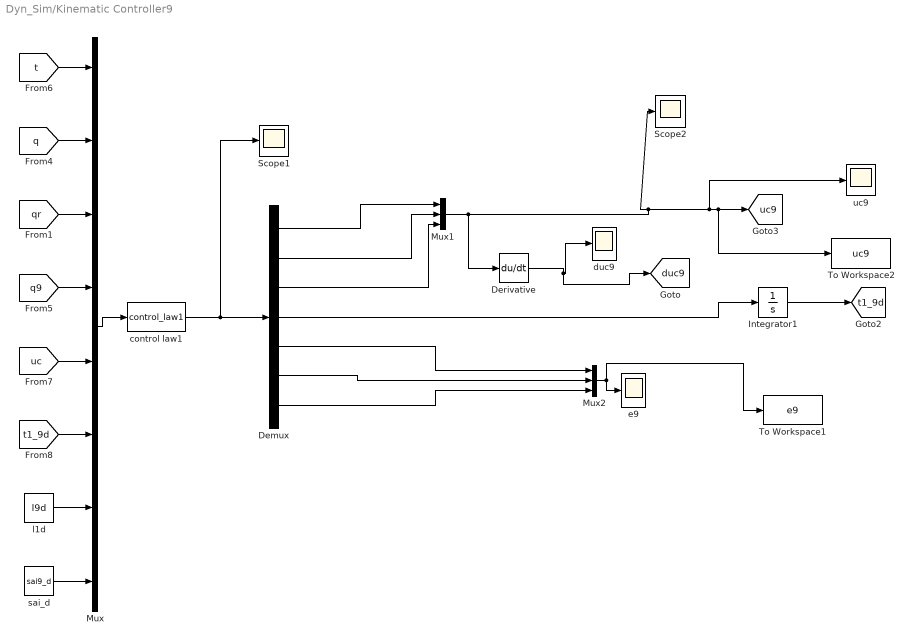
== system Dyn_Sim/Kinematic Controller9 ==
  Demux : Demux  Outputs=7
  Derivative : Derivative
  Integrator1 : Integrator  InitialCondition=pi/2
  Mux : Mux  Inputs=8
  Mux1 : Mux  Inputs=3
  Mux2 : Mux  Inputs=3
  Scope1 : Scope
  Scope2 : Scope
  To Workspace1 : ToWorkspace  VariableName=e9  SampleTime=-1
  To Workspace2 : ToWorkspace  VariableName=uc9  SampleTime=-1
  control law1 : MATLABFcn  MATLABFcn=control_law1  OutputDimensions=7  OutputSignalType=real
  duc9 : Scope
  e9 : Scope
  l1d : Constant  Value=l9d
  sai_d : Constant  Value=sai9_d
  "uc9 " : Scope
  tag scope: duc9=global, t1_9d=global, uc9=global
  wires:
  Demux/7 -> Mux2/3
  Demux/6 -> Mux2/2
  Demux/5 -> Mux2/1
  Demux/4 -> Integrator1/1
  Demux/3 -> Mux1/3
  sai_d/1 -> Mux/8
  l1d/1 -> Mux/7
  [t1_9d] -> Mux/6
  [t] -> Mux/1
  [q] -> Mux/2
  [qr] -> Mux/3
  [q9] -> Mux/4
  [uc] -> Mux/5
  Derivative/1 -> duc9/1, [duc9]
  Mux2/1 -> To Workspace1/1, e9/1
  Demux/2 -> Mux1/2
  Demux/1 -> Mux1/1
  Mux1/1 -> Scope2/1, [uc9], To Workspace2/1, "uc9 "/1, Derivative/1
  Integrator1/1 -> [t1_9d]
  Mux/1 -> control law1/1
  control law1/1 -> Demux/1, Scope1/1

== system Dyn_Sim/Kinematic Model1 ==
  Demux3 : Demux  Outputs=3
  Integrator1 : Integrator  InitialCondition=q0_1
  Mux3 : Mux  Inputs=2
  Scope3 : Scope
  Scope4 : Scope
  Scope6 : Scope
  To Workspace10 : ToWorkspace  VariableName=t1_1  SampleTime=-1
  To Workspace7 : ToWorkspace  VariableName=q1  SampleTime=-1
  To Workspace8 : ToWorkspace  VariableName=x1  SampleTime=-1
  To Workspace9 : ToWorkspace  VariableName=y1  SampleTime=-1
  kinematic_model : MATLABFcn  MATLABFcn=kinematic_model  OutputDimensions=3  OutputSignalType=real
  tag scope: q1=global
  wires:
  [q1] -> Mux3/1
  [uu1] -> Mux3/2
  Mux3/1 -> kinematic_model/1
  Demux3/3 -> Scope6/1, To Workspace10/1
  Demux3/1 -> Scope3/1, To Workspace8/1
  Demux3/2 -> Scope4/1, To Workspace9/1
  kinematic_model/1 -> Integrator1/1
  Integrator1/1 -> [q1], Demux3/1, To Workspace7/1

== system Dyn_Sim/Kinematic Model10 ==
  Demux3 : Demux  Outputs=3
  Integrator1 : Integrator  InitialCondition=q0_10
  Mux3 : Mux  Inputs=2
  Scope3 : Scope
  Scope4 : Scope
  Scope6 : Scope
  To Workspace10 : ToWorkspace  VariableName=t1_10  SampleTime=-1
  To Workspace7 : ToWorkspace  VariableName=q10  SampleTime=-1
  To Workspace8 : ToWorkspace  VariableName=x10  SampleTime=-1
  To Workspace9 : ToWorkspace  VariableName=y10  SampleTime=-1
  kinematic_model : MATLABFcn  MATLABFcn=kinematic_model  OutputDimensions=3  OutputSignalType=real
  tag scope: q10=global
  wires:
  Integrator1/1 -> To Workspace7/1, Demux3/1, [q10]
  kinematic_model/1 -> Integrator1/1
  Demux3/2 -> To Workspace9/1, Scope4/1
  Demux3/1 -> To Workspace8/1, Scope3/1
  Demux3/3 -> To Workspace10/1, Scope6/1
  Mux3/1 -> kinematic_model/1
  [uu10] -> Mux3/2
  [q10] -> Mux3/1

== system Dyn_Sim/Kinematic Model2 ==
  Demux3 : Demux  Outputs=3
  Integrator1 : Integrator  InitialCondition=q0_2
  Mux3 : Mux  Inputs=2
  Scope3 : Scope
  Scope4 : Scope
  Scope6 : Scope
  To Workspace10 : ToWorkspace  VariableName=t1_2  SampleTime=-1
  To Workspace7 : ToWorkspace  VariableName=q2  SampleTime=-1
  To Workspace8 : ToWorkspace  VariableName=x2  SampleTime=-1
  To Workspace9 : ToWorkspace  VariableName=y2  SampleTime=-1
  kinematic_model : MATLABFcn  MATLABFcn=kinematic_model  OutputDimensions=3  OutputSignalType=real
  tag scope: q2=global
  wires:
  Mux3/1 -> kinematic_model/1
  Demux3/2 -> To Workspace9/1, Scope4/1
  Demux3/1 -> To Workspace8/1, Scope3/1
  [q2] -> Mux3/1
  [uu2] -> Mux3/2
  kinematic_model/1 -> Integrator1/1
  Demux3/3 -> To Workspace10/1, Scope6/1
  Integrator1/1 -> To Workspace7/1, Demux3/1, [q2]

== system Dyn_Sim/Kinematic Model3 ==
  Demux3 : Demux  Outputs=3
  Integrator1 : Integrator  InitialCondition=q0_3
  Mux3 : Mux  Inputs=2
  Scope3 : Scope
  Scope4 : Scope
  Scope6 : Scope
  To Workspace10 : ToWorkspace  VariableName=t1_3  SampleTime=-1
  To Workspace7 : ToWorkspace  VariableName=q3  SampleTime=-1
  To Workspace8 : ToWorkspace  VariableName=x3  SampleTime=-1
  To Workspace9 : ToWorkspace  VariableName=y3  SampleTime=-1
  kinematic_model : MATLABFcn  MATLABFcn=kinematic_model  OutputDimensions=3  OutputSignalType=real
  tag scope: q3=global
  wires:
  [q3] -> Mux3/1
  [uu3] -> Mux3/2
  Mux3/1 -> kinematic_model/1
  Demux3/3 -> Scope6/1, To Workspace10/1
  Demux3/1 -> Scope3/1, To Workspace8/1
  Demux3/2 -> Scope4/1, To Workspace9/1
  kinematic_model/1 -> Integrator1/1
  Integrator1/1 -> [q3], Demux3/1, To Workspace7/1

== system Dyn_Sim/Kinematic Model4 ==
  Demux3 : Demux  Outputs=3
  Integrator1 : Integrator  InitialCondition=q0_4
  Mux3 : Mux  Inputs=2
  Scope3 : Scope
  Scope4 : Scope
  Scope6 : Scope
  To Workspace10 : ToWorkspace  VariableName=t1_4  SampleTime=-1
  To Workspace7 : ToWorkspace  VariableName=q4  SampleTime=-1
  To Workspace8 : ToWorkspace  VariableName=x4  SampleTime=-1
  To Workspace9 : ToWorkspace  VariableName=y4  SampleTime=-1
  kinematic_model : MATLABFcn  MATLABFcn=kinematic_model  OutputDimensions=3  OutputSignalType=real
  tag scope: q4=global
  wires:
  [q4] -> Mux3/1
  [uu4] -> Mux3/2
  Mux3/1 -> kinematic_model/1
  Demux3/3 -> Scope6/1, To Workspace10/1
  Demux3/1 -> Scope3/1, To Workspace8/1
  Demux3/2 -> Scope4/1, To Workspace9/1
  kinematic_model/1 -> Integrator1/1
  Integrator1/1 -> [q4], Demux3/1, To Workspace7/1

== system Dyn_Sim/Kinematic Model5 ==
  Demux3 : Demux  Outputs=3
  Integrator1 : Integrator  InitialCondition=q0_5
  Mux3 : Mux  Inputs=2
  Scope3 : Scope
  Scope4 : Scope
  Scope6 : Scope
  To Workspace10 : ToWorkspace  VariableName=t1_5  SampleTime=-1
  To Workspace7 : ToWorkspace  VariableName=q5  SampleTime=-1
  To Workspace8 : ToWorkspace  VariableName=x5  SampleTime=-1
  To Workspace9 : ToWorkspace  VariableName=y5  SampleTime=-1
  kinematic_model : MATLABFcn  MATLABFcn=kinematic_model  OutputDimensions=3  OutputSignalType=real
  tag scope: q5=global
  wires:
  [q5] -> Mux3/1
  [uu5] -> Mux3/2
  Mux3/1 -> kinematic_model/1
  Demux3/3 -> Scope6/1, To Workspace10/1
  Demux3/1 -> Scope3/1, To Workspace8/1
  Demux3/2 -> Scope4/1, To Workspace9/1
  kinematic_model/1 -> Integrator1/1
  Integrator1/1 -> [q5], Demux3/1, To Workspace7/1

== system Dyn_Sim/Kinematic Model6 ==
  Demux3 : Demux  Outputs=3
  Integrator1 : Integrator  InitialCondition=q0_6
  Mux3 : Mux  Inputs=2
  Scope3 : Scope
  Scope4 : Scope
  Scope6 : Scope
  To Workspace10 : ToWorkspace  VariableName=t1_6  SampleTime=-1
  To Workspace7 : ToWorkspace  VariableName=q6  SampleTime=-1
  To Workspace8 : ToWorkspace  VariableName=x6  SampleTime=-1
  To Workspace9 : ToWorkspace  VariableName=y6  SampleTime=-1
  kinematic_model : MATLABFcn  MATLABFcn=kinematic_model  OutputDimensions=3  OutputSignalType=real
  tag scope: q6=global
  wires:
  Integrator1/1 -> To Workspace7/1, Demux3/1, [q6]
  kinematic_model/1 -> Integrator1/1
  Demux3/2 -> To Workspace9/1, Scope4/1
  Demux3/1 -> To Workspace8/1, Scope3/1
  Demux3/3 -> To Workspace10/1, Scope6/1
  Mux3/1 -> kinematic_model/1
  [uu6] -> Mux3/2
  [q6] -> Mux3/1

== system Dyn_Sim/Kinematic Model7 ==
  Demux3 : Demux  Outputs=3
  Integrator1 : Integrator  InitialCondition=q0_7
  Mux3 : Mux  Inputs=2
  Scope3 : Scope
  Scope4 : Scope
  Scope6 : Scope
  To Workspace10 : ToWorkspace  VariableName=t1_7  SampleTime=-1
  To Workspace7 : ToWorkspace  VariableName=q7  SampleTime=-1
  To Workspace8 : ToWorkspace  VariableName=x7  SampleTime=-1
  To Workspace9 : ToWorkspace  VariableName=y7  SampleTime=-1
  kinematic_model : MATLABFcn  MATLABFcn=kinematic_model  OutputDimensions=3  OutputSignalType=real
  tag scope: q7=global
  wires:
  Integrator1/1 -> [q7], Demux3/1, To Workspace7/1
  Demux3/3 -> Scope6/1, To Workspace10/1
  kinematic_model/1 -> Integrator1/1
  [uu7] -> Mux3/2
  [q7] -> Mux3/1
  Demux3/1 -> Scope3/1, To Workspace8/1
  Demux3/2 -> Scope4/1, To Workspace9/1
  Mux3/1 -> kinematic_model/1

== system Dyn_Sim/Kinematic Model8 ==
  Demux3 : Demux  Outputs=3
  Integrator1 : Integrator  InitialCondition=q0_8
  Mux3 : Mux  Inputs=2
  Scope3 : Scope
  Scope4 : Scope
  Scope6 : Scope
  To Workspace10 : ToWorkspace  VariableName=t1_8  SampleTime=-1
  To Workspace7 : ToWorkspace  VariableName=q8  SampleTime=-1
  To Workspace8 : ToWorkspace  VariableName=x8  SampleTime=-1
  To Workspace9 : ToWorkspace  VariableName=y8  SampleTime=-1
  kinematic_model : MATLABFcn  MATLABFcn=kinematic_model  OutputDimensions=3  OutputSignalType=real
  tag scope: q8=global
  wires:
  Integrator1/1 -> To Workspace7/1, Demux3/1, [q8]
  kinematic_model/1 -> Integrator1/1
  Demux3/2 -> To Workspace9/1, Scope4/1
  Demux3/1 -> To Workspace8/1, Scope3/1
  Demux3/3 -> To Workspace10/1, Scope6/1
  Mux3/1 -> kinematic_model/1
  [uu8] -> Mux3/2
  [q8] -> Mux3/1

== system Dyn_Sim/Kinematic Model9 ==
  Demux3 : Demux  Outputs=3
  Integrator1 : Integrator  InitialCondition=q0_9
  Mux3 : Mux  Inputs=2
  Scope3 : Scope
  Scope4 : Scope
  Scope6 : Scope
  To Workspace10 : ToWorkspace  VariableName=t1_9  SampleTime=-1
  To Workspace7 : ToWorkspace  VariableName=q9  SampleTime=-1
  To Workspace8 : ToWorkspace  VariableName=x9  SampleTime=-1
  To Workspace9 : ToWorkspace  VariableName=y9  SampleTime=-1
  kinematic_model : MATLABFcn  MATLABFcn=kinematic_model  OutputDimensions=3  OutputSignalType=real
  tag scope: q9=global
  wires:
  Integrator1/1 -> To Workspace7/1, Demux3/1, [q9]
  kinematic_model/1 -> Integrator1/1
  Demux3/2 -> To Workspace9/1, Scope4/1
  Demux3/1 -> To Workspace8/1, Scope3/1
  Demux3/3 -> To Workspace10/1, Scope6/1
  Mux3/1 -> kinematic_model/1
  [uu9] -> Mux3/2
  [q9] -> Mux3/1

== system Dyn_Sim/Kinematic controller ==
  Demux1 : Demux  Outputs=3
  Demux2 : Demux  Outputs=6
  Derivative : Derivative
  Mux1 : Mux
  Mux2 : Mux  Inputs=2
  Mux3 : Mux  Inputs=3
  Mux4 : Mux  Inputs=3
  To Workspace5 : ToWorkspace  VariableName=u2c  SampleTime=-1
  To Workspace6 : ToWorkspace  VariableName=u1c  SampleTime=-1
  e : Scope
  kin cont : MATLABFcn  MATLABFcn=control_law  OutputDimensions=6  OutputSignalType=real
  tag scope: duc=global, uc=global
  wires:
  kin cont/1 -> Demux2/1
  Mux1/1 -> kin cont/1
  [t] -> Mux1/1
  Derivative/1 -> [duc]
  [qr] -> Mux1/3
  [q] -> Mux1/2
  [dqr] -> Mux1/4
  Demux1/3 -> To Workspace5/1
  Demux1/2 -> Mux2/2
  Demux1/1 -> Mux2/1
  Mux2/1 -> To Workspace6/1
  Demux2/4 -> Mux3/1
  Demux2/5 -> Mux3/2
  Demux2/6 -> Mux3/3
  Mux3/1 -> e/1
  Demux2/1 -> Mux4/1
  Demux2/2 -> Mux4/2
  Demux2/3 -> Mux4/3
  Mux4/1 -> Derivative/1, [uc], Demux1/1

== system Dyn_Sim/Kinematik model ==
  Demux3 : Demux  Outputs=3
  Integrator1 : Integrator  InitialCondition=q0
  Mux3 : Mux  Inputs=2
  Scope3 : Scope
  Scope4 : Scope
  Scope6 : Scope
  To Workspace10 : ToWorkspace  VariableName=phi  SampleTime=-1
  To Workspace7 : ToWorkspace  VariableName=q  SampleTime=-1
  To Workspace8 : ToWorkspace  VariableName=x  SampleTime=-1
  To Workspace9 : ToWorkspace  VariableName=y  SampleTime=-1
  kinematic_model : MATLABFcn  MATLABFcn=kinematic_model  OutputDimensions=3  OutputSignalType=real
  tag scope: phi=global, q=global
  wires:
  Integrator1/1 -> [q], Demux3/1, To Workspace7/1
  Demux3/2 -> Scope4/1, To Workspace9/1
  kinematic_model/1 -> Integrator1/1
  Demux3/3 -> [phi], Scope6/1, To Workspace10/1
  [uu] -> Mux3/2
  Mux3/1 -> kinematic_model/1
  [q] -> Mux3/1
  Demux3/1 -> Scope3/1, To Workspace8/1

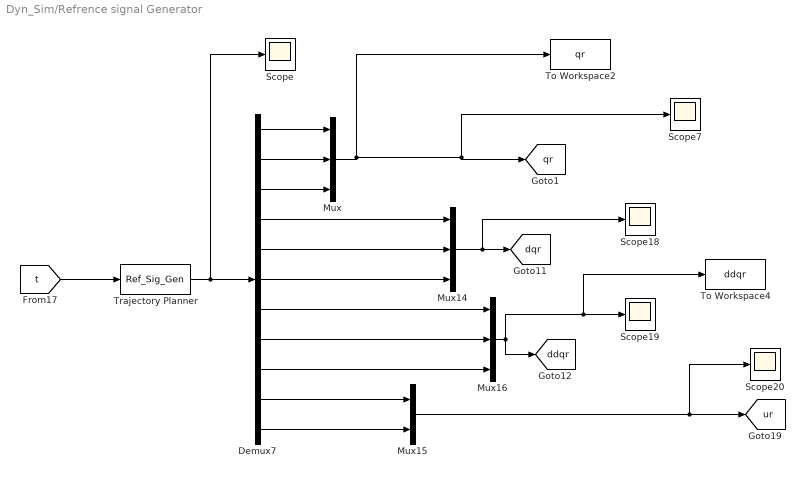
== system Dyn_Sim/Refrence signal Generator  ==
  Demux7 : Demux  Outputs=11
  Mux : Mux  Inputs=3
  Mux14 : Mux  Inputs=3
  Mux15 : Mux  Inputs=2
  Mux16 : Mux  Inputs=3
  Scope{,7,18..20} (5 alike) : Scope
  To Workspace2 : ToWorkspace  VariableName=qr  SampleTime=-1
      settings: Save2DSignal=2-D array (concatenate along first dimension)
  To Workspace4 : ToWorkspace  VariableName=ddqr  SampleTime=-1
      settings: Save2DSignal=2-D array (concatenate along first dimension)
  Trajectory Planner : MATLABFcn  MATLABFcn=Ref_Sig_Gen  OutputDimensions=11
  tag scope: ddqr=global, dqr=global, qr=global, ur=global
  wires:
  Trajectory Planner/1 -> Scope/1, Demux7/1
  Demux7/1 -> Mux/1
  [t] -> Trajectory Planner/1
  Demux7/9 -> Mux16/3
  Demux7/6 -> Mux14/3
  Mux15/1 -> Scope20/1, [ur]
  Demux7/5 -> Mux14/2
  Demux7/10 -> Mux15/1
  Demux7/2 -> Mux/2
  Demux7/3 -> Mux/3
  Mux16/1 -> [ddqr], To Workspace4/1, Scope19/1
  Demux7/7 -> Mux16/1
  Mux/1 -> To Workspace2/1, Scope7/1, [qr]
  Demux7/11 -> Mux15/2
  Mux14/1 -> Scope18/1, [dqr]
  Demux7/4 -> Mux14/1
  Demux7/8 -> Mux16/2

== system Dyn_Sim/dynamik model ==
  Demux1 : Demux  Outputs=3
  Integrator2 : Integrator  InitialCondition=u0
  Mux9 : Mux  Inputs=3
  To Workspace11 : ToWorkspace  VariableName=uu  SampleTime=-1
  dynamic_model : MATLABFcn  MATLABFcn=dynamic_model  OutputDimensions=3  OutputSignalType=real
  tag scope: duu=global, uu=global, vv=global
  wires:
  Demux1/2 -> [vv]
  Integrator2/1 -> To Workspace11/1, Demux1/1, [uu]
  [uu] -> Mux9/1
  [t] -> Mux9/3
  Mux9/1 -> dynamic_model/1
  dynamic_model/1 -> Integrator2/1, [duu]
  [tau] -> Mux9/2
